simulink model "InductionMotorScalarControlVSIOpenCircuitT3"  (R2015a)
settings: Solver=ode23s  StartTime=0.0  StopTime=10.0  MaxStep=1e-3  RelTol=1e-3
libraries: powerlib x10, simulink x3, powerlib_meascontrol x1
settings Model: Creator=range  LastModifiedBy=range

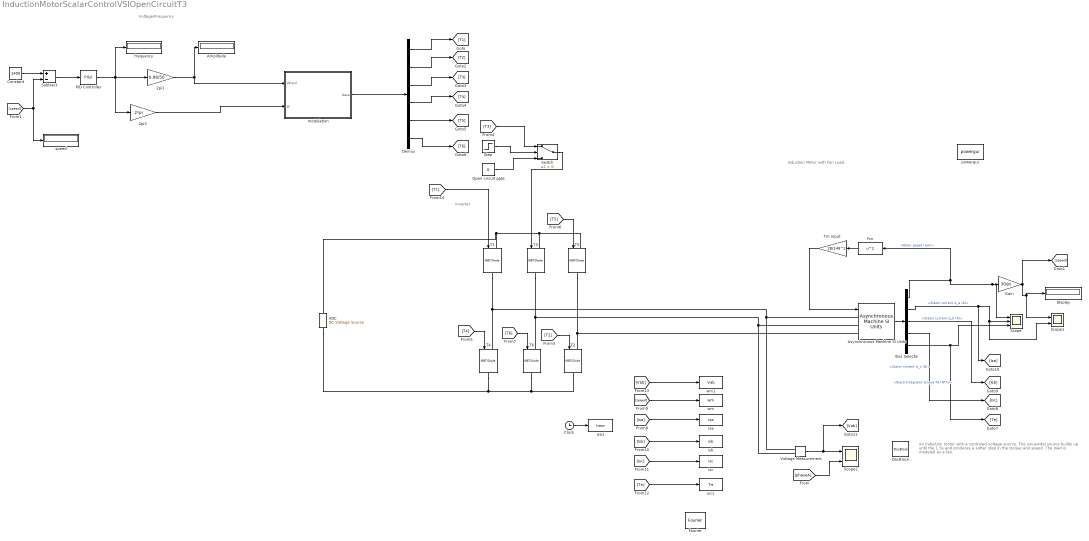
== system InductionMotorScalarControlVSIOpenCircuitT3 ==
  note: Inverter
  note: An induction motor with a controled voltage source.
      |
      | The sinusoidal source builds up until the 1.5s and
      | produces a softer step in the torque and speed.
      | The load is modeled as a fan.
  note: Induction Motor with Fan Load.
  note: Voltage/Frequency
  2pi1 : Gain  Gain=0.98/50
  2pi3 : Gain  Gain=2*pi
  Amplitude : Display
  Asynchronous Machine SI Units : powerlib/Machines/Asynchronous Machine SI Units  RotorType=Squirrel-cage  PresetModel="15:  5.4 HP (4KW)   400 V  50Hz 1430 RPM"  MechanicalLoad=Torque Tm  ShowDetailedParameters=on  ReferenceFrame=Rotor  Units=SI  MeasurementBus=off  NominalParameters=[4000 400 50]  Stator=[1.405 0.005839]  Rotor=[1.395 0.005839]  Cage1=[0.4155 0.002066]  Cage2=[0.4168 0.0003495]  Lm=0.1722  Mechanical=[0.0131 0.002985 2]  PolePairs=2  InitialConditions=[1 0 0 0 0 0 0 0]  SimulateSaturation=off  Saturation=[14.03593122, 27.81365428, 53.79336849, 72.68890987, 97.98006896, 148.6815601, 215.7428561, 302.9841135, 428.7778367 ; 230, 322, 414, 460, 506, 552, 598, 644, 690]  LoadFlowParameters=1492000  TsPowergui=0  TsBlock=-1  IterativeModel=Trapezoidal non iterative  Pmec=1.492e+006
  Bus Selector : BusSelector  OutputSignals=Mechanical.Rotor speed (wm),Stator measurements.Stator current is_a (A),Stator measurements.Stator current is_b (A),Stator measurements.Stator current is_c (A),Mechanical.Electromagnetic torque Te (N*m)
  Clock : Clock
  Constant : Constant  Value=1400
  Demux : Demux  Outputs=6
  Display : Display
  DocBlock : simulink/Model-Wide Utilities/DocBlock  DocumentType=Text
      content=|
      | Simulation of an induction motor connected to an inverter.
  Fcn : Fcn  Expr=u^2
  Fourier : powerlib_meascontrol/Measurements/Fourier  Freq=50  n=1  InInit=[0, 0]  Ts=0
  Gain : Gain  Gain=30/pi
  Open circuit gate : Constant  Value=0
  PID Controller : simulink/Continuous/PID Controller  Controller=PI  TimeDomain=Continuous-time  SampleTime=-1  IntegratorMethod=Forward Euler  FilterMethod=Forward Euler  Form=Parallel  UseFilter=on  ControllerParametersSource=internal  P=0.0001  I=0.09  D=0  N=100  InitialConditionSource=internal  InitialConditionForIntegrator=0  InitialConditionForFilter=0  ExternalReset=none  LimitOutput=on  UpperSaturationLimit=50  LowerSaturationLimit=-50  LinearizeAsGain=on  AntiWindupMode=clamping  Kb=1  TrackingMode=off  Kt=1  PParamMin=[]  PParamMax=[]  IParamMin=[]  IParamMax=[]  DParamMin=[]  DParamMax=[]  NParamMin=[]  NParamMax=[]  KbParamMin=[]  KbParamMax=[]  KtParamMin=[]  KtParamMax=[]  POutMin=[]  POutMax=[]  IOutMin=[]  IOutMax=[]  DOutMin=[]  DOutMax=[]  NOutMin=[]  NOutMax=[]  KbOutMin=[]  KbOutMax=[]  KtOutMin=[]  KtOutMax=[]  IntegratorOutMin=[]  IntegratorOutMax=[]  FilterOutMin=[]  FilterOutMax=[]  SumOutMin=[]  SumOutMax=[]  SumI1OutMin=[]  SumI1OutMax=[]  SumI2OutMin=[]  SumI2OutMax=[]  SumI3OutMin=[]  SumI3OutMax=[]  SumDOutMin=[]  SumDOutMax=[]  SaturationOutMin=[]  SaturationOutMax=[]  IntegratorContinuousStateAttributes=''  IntegratorStateMustResolveToSignalObject=off  IntegratorRTWStateStorageClass=Auto  FilterContinuousStateAttributes=''  FilterStateMustResolveToSignalObject=off  FilterRTWStateStorageClass=Auto  DifferentiatorICPrevScaledInput=0  DifferentiatorOutMin=[]  DifferentiatorOutMax=[]
  Scope : Scope  NumInputPorts=3
      settings: YMin=146.555~-12.5~25  YMax=146.62~12.5~30  MaxDataPoints=100000
  Scope1 : Scope  NumInputPorts=2
      settings: YMin=-5~-5  YMax=5~5
  Scope2 : Scope  NumInputPorts=2
      settings: YMin=-800~-1  YMax=800~1  SaveName=ScopeData2  MaxDataPoints=10000
  Step : Step  Time=5  Before=1  After=0  SampleTime=0
  Subtract : Sum  Inputs=+-
  Switch : Switch  Criteria=u2 > Threshold
  T{1..6} (6 alike) : powerlib/Power Electronics/IGBT//Diode  Ron=1e-3  Rs=1e5  Cs=inf  Measurements=off
  Tm input : Gain  Gain=28/149^2
  VDC : powerlib/Electrical Sources/DC Voltage Source  Amplitude=650  Measurements=None
  Voltage Measurement : powerlib/Measurements/Voltage Measurement  PhasorSimulation=off  OutputType=Complex  PSBequivalent=0
  frequency : Display
  isa : ToWorkspace  VariableName=isa  SampleTime=-1
  isa1 : ToWorkspace  VariableName=time  SampleTime=-1
  isb : ToWorkspace  VariableName=isb  SampleTime=-1
  isc : ToWorkspace  VariableName=isc  SampleTime=-1
  isc1 : ToWorkspace  VariableName=Te  SampleTime=-1
  modulation : Subsystem
  powergui : powerlib/powergui  Priority=1  SimulationMode=Discrete  SolverType=Tustin/Backward Euler (TBE)  SampleTime=1e-6  frequency=60  SPID=off  DisableSnubberDevices=off  DisableRonSwitches=off  DisableVfSwitches=off  SwTol=0  DisplayEquations=off  Interpol=off  methode=off  Ts=100  FunctionMessages=off  echomessages=off  HookPort=off  EnableUseOfTLC=off  x0status=blocks  frequencyindice=50  Pbase=100e6  ErrMax=1e-4  Iterations=50  UnitsV=kV  UnitsW=MW  buscounter=0  RestoreLinks=warning  ResistiveCurrentMeasurement=off  Frange=[0:2:500]  Ylog=off  Xlog=on  ShowGrid=off  save=off  variable=ZData  structure=0  ZoomFFT=off  StartTime=0.0  cycles=1  DisplayStyle=1  fundamental=60  FreqAxis=off  MaxFrequency=1000  frequencyindicesteady=1  RmsSteady=1  display=off
  speed : Display
  wm : ToWorkspace  VariableName=wm  SampleTime=-1
  wm1 : ToWorkspace  VariableName=Vab  SampleTime=-1
  wires:
  Asynchronous Machine SI Units/1 -> Bus Selector/1
  Bus Selector/1 -> Fcn/1, Scope/1, Gain/1  "<Rotor speed (wm)>"
  Bus Selector/2 -> [Isa], Scope1/2, Scope/2  "<Stator current is_a (A)>"
  Gain/1 -> Display/1, Scope1/1, [speed]
  Bus Selector/5 -> [Te], Scope/3  "<Electromagnetic torque Te (N*m)>"
  Tm input/1 -> Asynchronous Machine SI Units/1
  Fcn/1 -> Tm input/1
  Voltage Measurement/1 -> [Vab], Scope2/1
  [phaseA] -> Scope2/2
  2pi1/1 -> Amplitude/1, modulation/1(Vs(pu))
  Constant/1 -> Subtract/1
  [speed] -> speed/1, Subtract/2
  Subtract/1 -> PID Controller/1
  PID Controller/1 -> frequency/1, 2pi3/1, 2pi1/1
  2pi3/1 -> modulation/2(W)
  modulation/1(Gate) -> Demux/1
  Demux/6 -> [T6]
  Demux/1 -> [T1]
  Demux/2 -> [T2]
  Demux/3 -> [T3]
  Demux/4 -> [T4]
  Demux/5 -> [T5]
  [T5] -> T5/1
  [T4] -> T4/1
  [T2] -> T2/1
  [T6] -> T6/1
  [speed] -> wm/1
  [Isa] -> isa/1
  [Isb] -> isb/1
  [Isc] -> isc/1
  [Te] -> isc1/1
  Bus Selector/4 -> [Isc]  "<Stator current is_c (A)>"
  Bus Selector/3 -> [Isb]  "<Stator current is_b (A)>"
  [Vab] -> wm1/1
  Open circuit gate/1 -> Switch/3
  Step/1 -> Switch/2
  Clock/1 -> isa1/1
  Switch/1 -> T3/1
  [T3] -> Switch/1
  [T1] -> T1/1
  connections:
  Asynchronous Machine SI Units/LConn1 -- Voltage Measurement/LConn1 -- T1/RConn1 -- T4/LConn1
  T5/RConn1 -- Asynchronous Machine SI Units/LConn3 -- T2/LConn1
  T4/RConn1 -- VDC/LConn1 -- T6/RConn1 -- T2/RConn1
  Asynchronous Machine SI Units/LConn2 -- Voltage Measurement/LConn2 -- T3/RConn1 -- T6/LConn1
  T1/LConn1 -- VDC/RConn1 -- T3/LConn1 -- T5/LConn1

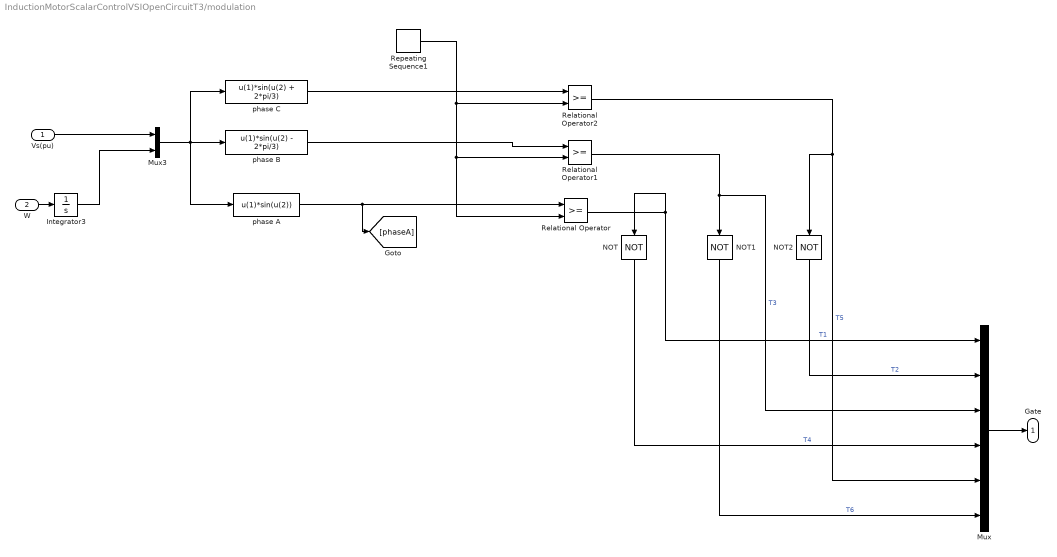
== system InductionMotorScalarControlVSIOpenCircuitT3/modulation ==
  Vs(pu) : Inport
  W : Inport  Port=2
  Integrator3 : Integrator
  Mux : Mux  Inputs=6
  Mux3 : Mux  Inputs=2
  NOT : Logic  Operator=NOT  AllPortsSameDT=off  OutDataTypeStr=boolean
  NOT1 : Logic  Operator=NOT  AllPortsSameDT=off  OutDataTypeStr=boolean
  NOT2 : Logic  Operator=NOT  AllPortsSameDT=off  OutDataTypeStr=boolean
  Relational Operator : RelationalOperator  OutDataTypeStr=boolean
  Relational Operator1 : RelationalOperator  OutDataTypeStr=boolean
  Relational Operator2 : RelationalOperator  OutDataTypeStr=boolean
  Repeating Sequence1 : simulink/Sources/Repeating Sequence  rep_seq_t=[0 (1/5000)/4 (2/5000)/4 (3/5000)/4 (4/5000)/4]  rep_seq_y=[0 1 0 -1 0]
  phase A : Fcn  Expr=u(1)*sin(u(2))
  phase B : Fcn  Expr=u(1)*sin(u(2) - 2*pi/3)
  phase C : Fcn  Expr=u(1)*sin(u(2) + 2*pi/3)
  Gate : Outport
  wires:
  Mux3/1 -> phase A/1, phase B/1, phase C/1
  W/1 -> Integrator3/1
  phase A/1 -> [phaseA], Relational Operator/1
  NOT/1 -> Mux/4  "T4"
  Relational Operator/1 -> Mux/1, NOT/1  "T1"
  phase C/1 -> Relational Operator2/1
  Relational Operator2/1 -> Mux/5, NOT2/1  "T5"
  phase B/1 -> Relational Operator1/1
  Relational Operator1/1 -> Mux/3, NOT1/1  "T3"
  NOT1/1 -> Mux/6  "T6"
  Repeating Sequence1/1 -> Relational Operator2/2, Relational Operator/2, Relational Operator1/2
  Vs(pu)/1 -> Mux3/1
  Integrator3/1 -> Mux3/2
  Mux/1 -> Gate/1
  NOT2/1 -> Mux/2  "T2"
